simulink model "velocity"  (Simulink 7.2)
settings: Solver=ode45  StartTime=0.0  StopTime=20  RelTol=1e-3
undefined symbols (not defined in the file): alpha, beta, Ki, Kp, Kt, Ts, w
settings Model: Creator=dnad  LastModifiedBy=dnad

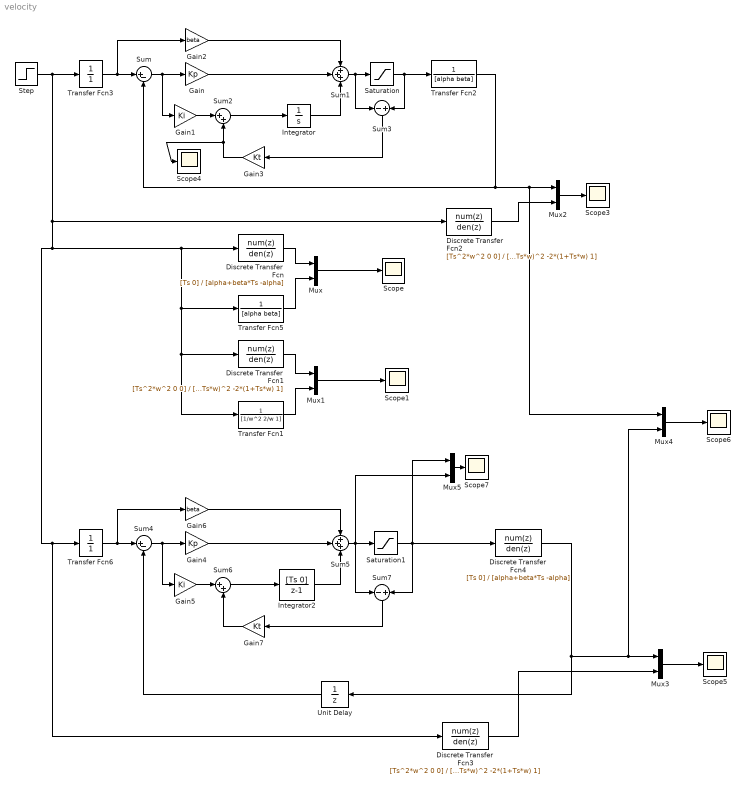
== system velocity ==
  Discrete Transfer Fcn : DiscreteTransferFcn  Numerator=[Ts 0]  Denominator=[alpha+beta*Ts -alpha]  SampleTime=Ts
  Discrete Transfer Fcn1 : DiscreteTransferFcn  Numerator=[Ts^2*w^2 0 0]  Denominator=[(1+Ts*w)^2 -2*(1+Ts*w) 1]  SampleTime=Ts
  Discrete Transfer Fcn2 : DiscreteTransferFcn  Numerator=[Ts^2*w^2 0 0]  Denominator=[(1+Ts*w)^2 -2*(1+Ts*w) 1]  SampleTime=Ts
  Discrete Transfer Fcn3 : DiscreteTransferFcn  Numerator=[Ts^2*w^2 0 0]  Denominator=[(1+Ts*w)^2 -2*(1+Ts*w) 1]  SampleTime=Ts
  Discrete Transfer Fcn4 : DiscreteTransferFcn  Numerator=[Ts 0]  Denominator=[alpha+beta*Ts -alpha]  SampleTime=Ts
  Gain : Gain  Gain=Kp  ParameterDataType=sfix(16)  ParameterScaling=2^0  OutDataType=sfix(16)  OutScaling=2^0
  Gain1 : Gain  Gain=Ki  ParameterDataType=sfix(16)  ParameterScaling=2^0  OutDataType=sfix(16)  OutScaling=2^0
  Gain2 : Gain  Gain=beta  ParameterDataType=sfix(16)  ParameterScaling=2^0  OutDataType=sfix(16)  OutScaling=2^0
  Gain3 : Gain  Orientation=left  Gain=Kt  ParameterDataType=sfix(16)  ParameterScaling=2^0  OutDataType=sfix(16)  OutScaling=2^0
  Gain4 : Gain  Gain=Kp  ParameterDataType=sfix(16)  ParameterScaling=2^0  OutDataType=sfix(16)  OutScaling=2^0
  Gain5 : Gain  Gain=Ki  ParameterDataType=sfix(16)  ParameterScaling=2^0  OutDataType=sfix(16)  OutScaling=2^0
  Gain6 : Gain  Gain=beta  ParameterDataType=sfix(16)  ParameterScaling=2^0  OutDataType=sfix(16)  OutScaling=2^0
  Gain7 : Gain  Orientation=left  Gain=Kt  ParameterDataType=sfix(16)  ParameterScaling=2^0  OutDataType=sfix(16)  OutScaling=2^0
  Integrator : Integrator
  Integrator2 : DiscreteTransferFcn  Numerator=[Ts 0]  Denominator=[1 -1]  SampleTime=Ts
  Mux{,1..5} (6 alike) : Mux  Inputs=2
  Saturation : Saturate  UpperLimit=20  LowerLimit=-20  OutDataType=sfix(16)  OutScaling=2^0
  Saturation1 : Saturate  UpperLimit=20  LowerLimit=-20  OutDataType=sfix(16)  OutScaling=2^0
  Scope{,1,3..7} (7 alike) : Scope
      Scope3 settings: SaveName=ScopeData3
      Scope4 settings: SaveName=ScopeData4
      Scope5 settings: SaveName=ScopeData5
      Scope6 settings: SaveName=ScopeData6
      Scope7 settings: SaveName=ScopeData7
  Step : Step  Time=120  Before=0.5  After=0  SampleTime=0
  Sum : Sum  Inputs=|+-  OutDataType=sfix(16)  OutScaling=2^0
  Sum1 : Sum  Inputs=+++  OutDataType=sfix(16)  OutScaling=2^0
  Sum2 : Sum  Inputs=|++  OutDataType=sfix(16)  OutScaling=2^0
  Sum3 : Sum  Orientation=down  Inputs=-+  OutDataType=sfix(16)  OutScaling=2^0
  Sum4 : Sum  Inputs=|+-  OutDataType=sfix(16)  OutScaling=2^0
  Sum5 : Sum  Inputs=+++  OutDataType=sfix(16)  OutScaling=2^0
  Sum6 : Sum  Inputs=|++  OutDataType=sfix(16)  OutScaling=2^0
  Sum7 : Sum  Orientation=down  Inputs=-+  OutDataType=sfix(16)  OutScaling=2^0
  Transfer Fcn1 : TransferFcn  Denominator=[1/w^2 2/w 1]
  Transfer Fcn2 : TransferFcn  Denominator=[alpha beta]
  Transfer Fcn3 : TransferFcn  Denominator=[1]
  Transfer Fcn5 : TransferFcn  Denominator=[alpha beta]
  Transfer Fcn6 : TransferFcn  Denominator=[1]
  Unit Delay : UnitDelay  Orientation=left  SampleTime=Ts
  wires:
  Sum/1 -> Gain/1, Gain1/1
  Step/1 -> Transfer Fcn3/1, Discrete Transfer Fcn2/1, Discrete Transfer Fcn/1, Transfer Fcn5/1, Discrete Transfer Fcn1/1, Transfer Fcn1/1, Transfer Fcn6/1, Discrete Transfer Fcn3/1
  Sum1/1 -> Sum3/1, Saturation/1
  Mux/1 -> Scope/1
  Gain/1 -> Sum1/2
  Transfer Fcn3/1 -> Sum/1, Gain2/1
  Gain1/1 -> Sum2/1
  Saturation/1 -> Transfer Fcn2/1, Sum3/2
  Sum3/1 -> Gain3/1
  Sum2/1 -> Integrator/1
  Integrator/1 -> Sum1/3
  Gain3/1 -> Scope4/1, Sum2/2
  Transfer Fcn2/1 -> Sum/2, Mux2/1, Mux4/1
  Discrete Transfer Fcn/1 -> Mux/1
  Transfer Fcn5/1 -> Mux/2
  Discrete Transfer Fcn1/1 -> Mux1/1
  Transfer Fcn1/1 -> Mux1/2
  Mux1/1 -> Scope1/1
  Mux2/1 -> Scope3/1
  Discrete Transfer Fcn2/1 -> Mux2/2
  Sum4/1 -> Gain4/1, Gain5/1
  Sum5/1 -> Mux5/2, Saturation1/1, Sum7/1
  Gain4/1 -> Sum5/2
  Transfer Fcn6/1 -> Sum4/1, Gain6/1
  Gain5/1 -> Sum6/1
  Sum7/1 -> Gain7/1
  Sum6/1 -> Integrator2/1
  Integrator2/1 -> Sum5/3
  Gain6/1 -> Sum5/1
  Discrete Transfer Fcn4/1 -> Mux3/1, Mux4/2, Unit Delay/1
  Mux3/1 -> Scope5/1
  Discrete Transfer Fcn3/1 -> Mux3/2
  Mux4/1 -> Scope6/1
  Gain2/1 -> Sum1/1
  Saturation1/1 -> Mux5/1, Sum7/2, Discrete Transfer Fcn4/1
  Unit Delay/1 -> Sum4/2
  Mux5/1 -> Scope7/1
  Gain7/1 -> Sum6/2
